simulink model "Control_model_10DOF_fin"  (R2016b)
settings: Solver=FixedStepAuto  StartTime=0.0  StopTime=10  FixedStep=0.0001  RelTol=1e-3
InitFcn:
  | Initialisation_ctr_10DOF_fin
values from neighbouring files (symbols this model uses):
  COM_Parameters = [-lpelvis/2;r2;0]    [Initialisation_ctr_10DOF_fin.m]
  DH_Parameters = [hfoot 0 ... (first row only)    [Initialisation_ctr_10DOF_fin.m]
  dTrunk = trunklbd(3)    [Initialisation_ctr_10DOF_fin.m]
  dxFootSM = dxFoot    [Initialisation_ctr_10DOF_fin.m]
  dxTrunk = 0.1    [Initialisation_ctr_10DOF_fin.m]
  Foot_Parameters = [0;-(lFoot/2-lHeel);0]    [Initialisation_ctr_10DOF_fin.m]
  HAA2HEE = [0; 0; 0.001]    [Initialisation_ctr_10DOF_fin.m]
  HEE2HFE = 0.5*[0.2; 0; 0]    [Initialisation_ctr_10DOF_fin.m]
  height_vrp = CoM_position(1)    [Initialisation_ctr_10DOF_fin.m]
  hTrunk = trunklbd(1)    [Initialisation_ctr_10DOF_fin.m]
  initial_CoM_position = R*CoM_position    [Initialisation_ctr_10DOF_fin.m]
  initial_CoM_velocity = [0;0;0]    [Initialisation_ctr_10DOF_fin.m]
  initial_left_foot = [0;0;-stance_width/2]    [Initialisation_ctr_10DOF_fin.m]
  initial_right_foot = [0;0;stance_width/2]    [Initialisation_ctr_10DOF_fin.m]
  initial_RorL = 0    [Initialisation_ctr_10DOF_fin.m]
  jointsinitial = [9;-15;6;0;0;6;-15;9]/180*pi    [Initialisation_ctr_10DOF_fin.m]
  K_DCM = 4.3*[1 0 0 ... (first row only)    [Initialisation_ctr_10DOF_fin.m]
  kD_left = mbody*[0.95 0 0 0 ... (first row only)    [Initialisation_ctr_10DOF_fin.m]
  kD_right = mbody*[0.12 0 0 0 ... (first row only)    [Initialisation_ctr_10DOF_fin.m]
  kI_left = mbody*[35 0 0 0 ... (first row only)    [Initialisation_ctr_10DOF_fin.m]
  kI_right = mbody*[38.2 0 0 0 ... (first row only)    [Initialisation_ctr_10DOF_fin.m]
  kP_left = mbody*[75 0 0 0 ... (first row only)    [Initialisation_ctr_10DOF_fin.m]
  kP_right = mbody*[5.6 0 0 0 ... (first row only)    [Initialisation_ctr_10DOF_fin.m]
  Lenght = [lShank;lThigh]    [Initialisation_ctr_10DOF_fin.m]
  lFootSM = lFoot    [Initialisation_ctr_10DOF_fin.m]
  lpelvis = wPelvis    [Initialisation_ctr_10DOF_fin.m]
  mass = mbody    (= 60)    [Initialisation_ctr_10DOF_fin.m]
  Masses = [mThigh; mShank; mTrunk]    [Initialisation_ctr_10DOF_fin.m]
  nb_step = 4    [Initialisation_ctr_10DOF_fin.m]
  nb_step_pattern = 20    [Initialisation_ctr_10DOF_fin.m]
  Pelvis_Parameters = [-lpelvis/2;hTrunk/2;0]    [Initialisation_ctr_10DOF_fin.m]
  stance_width = lpelvis    [Initialisation_ctr_10DOF_fin.m]
  stride_lenght = 0.50    (= 0.5)    [Initialisation_ctr_10DOF_fin.m]
  T_DS = time_DS    (= 0.4)    [Initialisation_ctr_10DOF_fin.m]
  T_IT = time_DS    (= 0.4)    [Initialisation_ctr_10DOF_fin.m]
  T_SS = time_swing    (= 1.6)    [Initialisation_ctr_10DOF_fin.m]
  time_DS = (time_stance-time_swing)/2    (= 0.4)    [Initialisation_ctr_10DOF_fin.m]
  time_stance = 60/100*time_stride    (= 2.4)    [Initialisation_ctr_10DOF_fin.m]
  time_step = time_stride/2    (= 2)    [Initialisation_ctr_10DOF_fin.m]
  time_swing = 40/100*time_stride    (= 1.6)    [Initialisation_ctr_10DOF_fin.m]
  validity_angle = [-20*pi/180 20*pi/180 ... (first row only)    [Initialisation_ctr_10DOF_fin.m]
  wTrunk = trunklbd(2)    [Initialisation_ctr_10DOF_fin.m]
  x4CoM = CoM_position(1)-XR4(1)    [Initialisation_ctr_10DOF_fin.m]
undefined symbols (not defined in the file or in its folder): dsegment, hFoot, l, lFoot, omega0_x, omega0_z, rho, wPelvis, X, Xp_x, Xp_z, Y, Z
undefined symbols (not defined in the file): k_grf, lShankSM, lThighSM, mShank, mThigh
libraries: nesl_utility x247, sm_lib x215, dspindex x12, FootPlacementLibrary x8, dspsigops x4, dspswit3 x1
(part 18 of 18)

== stateflow chart Control_model_10DOF_fin/Time//State Machine/Chart ==
  state DS_Transfert_Left
    entry: State=4;
    RorL=true;
  state Initial_Transfert_Right
    entry: State=1;
    RorL=false;
  state SS_Left_Swing
    entry: State=2;
    RorL=false;
  state Finish_Left_swing
    entry: State=3;
    RorL=false;
  state Stance
    entry: State=0;
  state Initial_Transfert_Left
    entry: State=1;
    RorL=true;
  state SS_Right_Swing
    entry: State=2;
    RorL=true;
  state DS_Transfert_Right
    entry: State=4;
    RorL=false;
  state Finish_Right_swing
    entry: State=3;
    RorL=true;
  DS_Transfert_Right -> SS_Left_Swing : [t>=T_DS]
  SS_Left_Swing -> DS_Transfert_Left [order 1] : [t>=T_SS && L_contact==1]
  Stance -> Initial_Transfert_Right [order 1] : [initial_RorL==0]
  DS_Transfert_Left -> SS_Right_Swing : [t>=T_DS]
  Finish_Left_swing -> DS_Transfert_Left : [L_contact==1]
  Initial_Transfert_Right -> SS_Left_Swing : [t>=T_IT]
  SS_Left_Swing -> Finish_Left_swing [order 2] : [t>=T_SS && L_contact==0]
  (default) -> Stance
  Stance -> Initial_Transfert_Left [order 2] : [initial_RorL==1]
  SS_Right_Swing -> DS_Transfert_Right [order 1] : [t>=T_SS && R_contact==1]
  Initial_Transfert_Left -> SS_Right_Swing : [t>=T_IT]
  SS_Right_Swing -> Finish_Right_swing [order 2] : [t>=T_SS && R_contact==0]
  Finish_Right_swing -> DS_Transfert_Right : [R_contact==1]
  data: t input; R_contact input; initial_RorL parameter; L_contact input; State output; RorL output boolean size=1; T_DS parameter; T_SS parameter; T_IT parameter

== matlab function Control_model_10DOF_fin/Trajectory generator/DCM trajectory/DS/DCM estimate fin ==
  data: r_vrp input double size=3; DCM_position output double size=3; DCM_velocity output double size=3; r_DCM input double size=3; time_stance parameter double size=1; height_vrp parameter double size=1; time input double size=1
 function [DCM_position,DCM_velocity] = DCM_trajectory_generator_DS(r_vrp,r_DCM,time_stance, height_vrp,time)

%gravity
g=9.81;

% r_vrp(2)=r_vrp(2)/2;
% r_DCM(2)=r_DCM(2)/2;

%% DCM Trajectory

DCM_position=r_vrp+exp(sqrt(g/height_vrp)*(time-time_stance))*(r_DCM-r_vrp);
DCM_velocity=sqrt(g/height_vrp)*exp(sqrt(g/height_vrp)*(time-time_stance))*(r_DCM-r_vrp);

== matlab function Control_model_10DOF_fin/Trajectory generator/DCM trajectory/DS/DCM_points_position ==
  data: feet_positions input double; r_vrp output double size=3*(nb_step-1); r_DCM output double size=3*(nb_step-2); height_vrp parameter size=1; time_step parameter size=1; nb_step parameter size=1; Foot_Parameters parameter
function [r_vrp,r_DCM] =  Point_positions(feet_positions,height_vrp, time_step,nb_step,Foot_Parameters )

for i=1:3:length(feet_positions)
    feet_positions(i:(i+2))=feet_positions(i:(i+2));%+Foot_Parameters;
end

%gravity
g=9.81;

r_vrp=zeros(3*(nb_step-1),1);
r_DCM=zeros(3*(nb_step-2),1);

%Virtual Repellent Point position
for i=1:(nb_step-1)
    r_vrp((3*(i-1)+1):(3*i),1)=feet_positions((3*(i)+1):(3*(i+1)),1)+[0;height_vrp;0];
end

%final DCM position
r_DCM((3*((nb_step-2)-1)+1):(3*(nb_step-2)),1)=r_vrp((3*(nb_step-2)+1):(3*(nb_step-1)),1);

%%DCM point creation
for i=nb_step-3:-1:1
    r_DCM(3*(i-1)+1:(3*i),1)=r_vrp(3*(i)+1:(3*(i+1)),1)+exp(-sqrt(g/height_vrp)*time_step)*(r_DCM(3*(i)+1:(3*(i+1)),1)-r_vrp((3*(i)+1):(3*(i+1))));
end

== matlab function Control_model_10DOF_fin/Trajectory generator/DCM trajectory/DS/MATLAB Function ==
  data: DCM_position_ini input; DCM_position output; DCM_velocity_ini input; DCM_position_fin input; DCM_velocity_fin input; DCM_velocity output; time input; time_DS parameter size=1
function [DCM_position,DCM_velocity] = Polynomial_interpolation(DCM_position_ini,DCM_velocity_ini,DCM_position_fin,DCM_velocity_fin,time, time_DS)

P=[2/time_DS^3 1/time_DS^2 -2/time_DS^3 1/time_DS^2;
    -3/time_DS^2 -2/time_DS 3/time_DS^2 -1/time_DS;
    0 1 0 0;
    1 0 0 0];
P=P*[DCM_position_ini';
    DCM_velocity_ini';
    DCM_position_fin';
    DCM_velocity_fin'];

 T=[time^3 time^2 time 1;
     3*time^2 2*time 1 0];
 
 Res=T*P;
 
 DCM_position=[Res(1,1);Res(1,2);Res(1,3)];
 DCM_velocity=[Res(2,1);Res(2,2);Res(2,3)];

end

== matlab function Control_model_10DOF_fin/Trajectory generator/DCM trajectory/Finish_swing_phase//SS/DCM trajectory generator ==
  data: r_vrp input double size=3; DCM_position output double size=3; DCM_velocity output double size=3; r_DCM input double size=3; time_stance parameter double size=1; height_vrp parameter double size=1; time input double size=1
function [DCM_position,DCM_velocity] = DCM_trajectory_generator(r_vrp,r_DCM,time_stance, height_vrp,time)

%gravity
g=9.81;

% r_vrp(2)=r_vrp(2)/2;
% r_DCM(2)=r_DCM(2)/2;

%% DCM Trajectory

DCM_position=r_vrp+exp(sqrt(g/height_vrp)*(time-time_stance))*(r_DCM-r_vrp);
DCM_velocity=sqrt(g/height_vrp)*exp(sqrt(g/height_vrp)*(time-time_stance))*(r_DCM-r_vrp);

== matlab function Control_model_10DOF_fin/Trajectory generator/DCM trajectory/Finish_swing_phase//SS/DCM_points_position ==
  data: feet_positions input double; r_vrp output double size=3*(nb_step-1); r_DCM output double size=3*(nb_step-2); height_vrp parameter size=1; time_step parameter size=1; nb_step parameter size=1; Foot_Parameters parameter
function [r_vrp,r_DCM] =  Point_positions(feet_positions,height_vrp, time_step,nb_step,Foot_Parameters )

for i=1:3:length(feet_positions)
    feet_positions(i:(i+2))=feet_positions(i:(i+2));%+Foot_Parameters;
end

%gravity
g=9.81;

r_vrp=zeros(3*(nb_step-1),1);
r_DCM=zeros(3*(nb_step-2),1);

%Virtual Repellent Point position
for i=1:(nb_step-1)
    r_vrp((3*(i-1)+1):(3*i),1)=feet_positions((3*(i)+1):(3*(i+1)),1)+[0;height_vrp;0];
end

%final DCM position
r_DCM((3*((nb_step-2)-1)+1):(3*(nb_step-2)),1)=r_vrp((3*(nb_step-2)+1):(3*(nb_step-1)),1);

%%DCM point creation
for i=nb_step-3:-1:1
    r_DCM(3*(i-1)+1:(3*i),1)=r_vrp(3*(i)+1:(3*(i+1)),1)+exp(-sqrt(g/height_vrp)*time_step)*(r_DCM(3*(i)+1:(3*(i+1)),1)-r_vrp((3*(i)+1):(3*(i+1))));
end

== matlab function Control_model_10DOF_fin/Trajectory generator/DCM trajectory/Initial_Transfert/DCM_estimate_fin/DCM trajectory generator ==
  data: r_vrp input double size=3; DCM_position output double size=3; DCM_velocity output double size=3; r_DCM input double size=3; time_stance parameter double size=1; height_vrp parameter double size=1; time input double size=1
 function [DCM_position,DCM_velocity] = DCM_trajectory_generator_DS(r_vrp,r_DCM,time_stance, height_vrp,time)

%gravity
g=9.81;

% r_vrp(2)=r_vrp(2)/2;
% r_DCM(2)=r_DCM(2)/2;

%% DCM Trajectory

DCM_position=r_vrp+exp(sqrt(g/height_vrp)*(time-time_stance))*(r_DCM-r_vrp);
DCM_velocity=sqrt(g/height_vrp)*exp(sqrt(g/height_vrp)*(time-time_stance))*(r_DCM-r_vrp);

== matlab function Control_model_10DOF_fin/Trajectory generator/DCM trajectory/Initial_Transfert/DCM_points_position ==
  data: feet_positions input double; r_vrp output double size=3*(nb_step-1); r_DCM output double size=3*(nb_step-2); height_vrp parameter size=1; time_step parameter size=1; nb_step parameter size=1; Foot_Parameters parameter
function [r_vrp,r_DCM] =  Point_positions(feet_positions,height_vrp, time_step,nb_step,Foot_Parameters )

for i=1:3:length(feet_positions)
    feet_positions(i:(i+2))=feet_positions(i:(i+2));%+Foot_Parameters;
end

%gravity
g=9.81;

r_vrp=zeros(3*(nb_step-1),1);
r_DCM=zeros(3*(nb_step-2),1);

%Virtual Repellent Point position
for i=1:(nb_step-1)
    r_vrp((3*(i-1)+1):(3*i),1)=feet_positions((3*(i)+1):(3*(i+1)),1)+[0;height_vrp;0];
end

%final DCM position
r_DCM((3*((nb_step-2)-1)+1):(3*(nb_step-2)),1)=r_vrp((3*(nb_step-2)+1):(3*(nb_step-1)),1);

%%DCM point creation
for i=nb_step-3:-1:1
    r_DCM(3*(i-1)+1:(3*i),1)=r_vrp(3*(i)+1:(3*(i+1)),1)+exp(-sqrt(g/height_vrp)*time_step)*(r_DCM(3*(i)+1:(3*(i+1)),1)-r_vrp((3*(i)+1):(3*(i+1))));
end

== matlab function Control_model_10DOF_fin/Trajectory generator/DCM trajectory/Initial_Transfert/MATLAB Function ==
  data: DCM_position_ini input; DCM_position output; DCM_velocity_ini input; DCM_position_fin input; DCM_velocity_fin input; DCM_velocity output; time input; T_IT parameter size=1
function [DCM_position,DCM_velocity] = Polynomial_interpolation(DCM_position_ini,DCM_velocity_ini,DCM_position_fin,DCM_velocity_fin,time, T_IT)

P=[2/T_IT^3 1/T_IT^2 -2/T_IT^3 1/T_IT^2;
    -3/T_IT^2 -2/T_IT 3/T_IT^2 -1/T_IT;
    0 1 0 0;
    1 0 0 0];
P=P*[DCM_position_ini';
    DCM_velocity_ini';
    DCM_position_fin';
    DCM_velocity_fin'];

 T=[time^3 time^2 time 1;
     3*time^2 2*time 1 0];
 
 Res=T*P;
 
 DCM_position=[Res(1,1);Res(1,2);Res(1,3)];
 DCM_velocity=[Res(2,1);Res(2,2);Res(2,3)];

end

== matlab function Control_model_10DOF_fin/Trajectory generator/Enabled and Triggered Subsystem 1/Feet Pattern generator/Pattern creator ==
  data: swing_foot_position input size=[3 1]; stance_foot_position input double size=3; feet_positions output double size=3*(nb_step_pattern); RorL input size=1; nb_step_pattern parameter single size=1; stride_lenght parameter double size=1; stance_width parameter single size=1
  function feet_positions  = pattern_creator(swing_foot_position,stance_foot_position,RorL,nb_step_pattern,stride_lenght,stance_width)

feet_positions=zeros(3*(nb_step_pattern),1);


feet_positions(1:3,1)=swing_foot_position(:);
feet_positions(4:6,1)=stance_foot_position(:);
if RorL==true
    feet_positions(7:9,1)=stance_foot_position(:)+[stride_lenght/2;0;stance_width];
    if nb_step_pattern==4
        feet_positions(10:12,1)=feet_positions(7:9,1)+[0;0;-stance_width];
    end
else
    feet_positions(7:9,1)=stance_foot_position(:)+[stride_lenght/2;0;-stance_width];
    if nb_step_pattern==4
        feet_positions(10:12,1)=feet_positions(7:9,1)+[0;0;stance_width];
    end
end

if nb_step_pattern>4
    for i=4:nb_step_pattern-1
        if i==nb_step_pattern
            feet_positions((3*(i-1)+1):(3*i),1)=feet_positions((3*(i-3)+1):(3*(i-2)),1)+[stride_lenght/2;0;0];
        else
            feet_positions((3*(i-1)+1):(3*i),1)=feet_positions((3*(i-3)+1):(3*(i-2)),1)+[stride_lenght;0;0];
        end
        if i~=nb_step_pattern
            if i+1==nb_step_pattern
                feet_positions((3*i+1):(3*(i+1)),1)=feet_positions((3*(i-2)+1):(3*(i-1)),1)+[stride_lenght/2;0;0];
            else
                feet_positions((3*i+1):(3*(i+1)),1)=feet_positions((3*(i-2)+1):(3*(i-1)),1)+[stride_lenght;0;0];
            end
        end
    end
end

== matlab function Control_model_10DOF_fin/Trajectory generator/Enabled and Triggered Subsystem 1/initial position1/Left/MATLAB Function ==
  data: T input; X output
function X = fcn(T)

X=T(1:3,4);
X(2)=0;

== matlab function Control_model_10DOF_fin/Trajectory generator/Enabled and Triggered Subsystem 1/initial position1/Left/MATLAB Function1 ==
  data: T input; X output
function X = fcn(T)

X=T(1:3,4);
X(2)=0;

== matlab function Control_model_10DOF_fin/Trajectory generator/Enabled and Triggered Subsystem 1/initial position1/Right/MATLAB Function ==
  data: T input; X output
function X = fcn(T)

X=T(1:3,4);
X(2)=0;

== matlab function Control_model_10DOF_fin/Trajectory generator/Enabled and Triggered Subsystem 1/initial position1/Right/MATLAB Function1 ==
  data: T input; X output
function X = fcn(T)

X=T(1:3,4);
X(2)=0;

== matlab function Control_model_10DOF_fin/Trajectory generator/Enabled and Triggered Subsystem 1/initial position2/Left/MATLAB Function ==
  data: T input; X output
function X = fcn(T)

X=T(1:3,4);
X(2)=0;

== matlab function Control_model_10DOF_fin/Trajectory generator/Enabled and Triggered Subsystem 1/initial position2/Left/MATLAB Function1 ==
  data: T input; X output
function X = fcn(T)

X=T(1:3,4);
X(2)=0;

== matlab function Control_model_10DOF_fin/Trajectory generator/Enabled and Triggered Subsystem 1/initial position2/Right/MATLAB Function ==
  data: T input; X output
function X = fcn(T)

X=T(1:3,4);
X(2)=0;

== matlab function Control_model_10DOF_fin/Trajectory generator/Enabled and Triggered Subsystem 1/initial position2/Right/MATLAB Function1 ==
  data: T input; X output
function X = fcn(T)

X=T(1:3,4);
X(2)=0;

== matlab function Control_model_10DOF_fin/Trajectory generator/Hip trajectory2/DS/Hip trajectory ==
  data: current_time input; hip_angle_des output double size=1; time_DS parameter double size=1
function hip_angle_des= hip_trajectory(current_time, time_DS)


%% knee trajectory

knee_angle_ini=0;
knee_angle_fin=-3.3*pi/180;

slope_ini=0; 
slope_fin=0;

% current_time=current_time;
% 
% knee_angle_des=knee_angle_ini+slope_ini*current_time+(3*(knee_angle_fin-knee_angle_ini)-2*slope_ini-slope_fin)*(current_time)^2+(2*(knee_angle_ini-knee_angle_fin)+slope_ini+slope_fin)*(current_time)^3;

P=[2/(time_DS)^3 1/(time_DS)^2 -2/(time_DS)^3 1/(time_DS)^2;
    -3/(time_DS)^2 -2/(time_DS) 3/(time_DS)^2 -1/(time_DS);
    0 1 0 0;
    1 0 0 0];
P=P*[knee_angle_ini;
    slope_ini;
    knee_angle_fin;
    slope_fin];

 time_DS=[current_time^3 current_time^2 current_time 1;
     3*current_time^2 2*current_time 1 0];
 
 Res=time_DS*P;
 
 hip_angle_des=Res(1,1);

== matlab function Control_model_10DOF_fin/Trajectory generator/Hip trajectory2/Initial_Transfert/Hip trajectory ==
  data: current_time input; time_DS parameter double size=1; hip_angle_des output double size=1
function hip_angle_des= hip_trajectory(current_time, time_DS)


%% knee trajectory

knee_angle_ini=0;
knee_angle_fin=-3.3*pi/180;

slope_ini=0; 
slope_fin=0;

% current_time=current_time;
% 
% knee_angle_des=knee_angle_ini+slope_ini*current_time+(3*(knee_angle_fin-knee_angle_ini)-2*slope_ini-slope_fin)*(current_time)^2+(2*(knee_angle_ini-knee_angle_fin)+slope_ini+slope_fin)*(current_time)^3;

P=[2/(time_DS)^3 1/(time_DS)^2 -2/(time_DS)^3 1/(time_DS)^2;
    -3/(time_DS)^2 -2/(time_DS) 3/(time_DS)^2 -1/(time_DS);
    0 1 0 0;
    1 0 0 0];
P=P*[knee_angle_ini;
    slope_ini;
    knee_angle_fin;
    slope_fin];

 T=[current_time^3 current_time^2 current_time 1;
     3*current_time^2 2*current_time 1 0];
 
 Res=T*P;
 
 hip_angle_des=Res(1,1);

== matlab function Control_model_10DOF_fin/Trajectory generator/Hip trajectory2/SS/Subsystem2/Subsystem/Hip trajectory ==
  data: current_time input; time_swing parameter double size=1; hip_angle_des output double size=1
function hip_angle_des= hip_trajectory(current_time, time_swing)


%% knee trajectory

knee_angle_ini=-3.3*pi/180;
knee_angle_fin=0;

slope_ini=0; 
slope_fin=0;

% current_time=current_time;
% 
% knee_angle_des=knee_angle_ini+slope_ini*current_time+(3*(knee_angle_fin-knee_angle_ini)-2*slope_ini-slope_fin)*(current_time)^2+(2*(knee_angle_ini-knee_angle_fin)+slope_ini+slope_fin)*(current_time)^3;

P=[2/(time_swing/2)^3 1/(time_swing/2)^2 -2/(time_swing/2)^3 1/(time_swing/2)^2;
    -3/(time_swing/2)^2 -2/(time_swing/2) 3/(time_swing/2)^2 -1/(time_swing/2);
    0 1 0 0;
    1 0 0 0];
P=P*[knee_angle_ini;
    slope_ini;
    knee_angle_fin;
    slope_fin];

 T=[current_time^3 current_time^2 current_time 1;
     3*current_time^2 2*current_time 1 0];
 
 Res=T*P;
 
 hip_angle_des=Res(1,1);

== matlab function Control_model_10DOF_fin/Trajectory generator/Subsystem1/SS/Swing foot trajectory ==
  data: Swing_foot_position_des output; foot_position_ini input; foot_position_fin input; time input double size=1; time_swing parameter double size=1
function Swing_foot_position_des  = Polynomial_interpolation(foot_position_ini,foot_position_fin,time, time_swing)

P=[2/(time_swing)^3 1/(time_swing)^2 -2/(time_swing)^3 1/(time_swing)^2;
    -3/(time_swing)^2 -2/(time_swing) 3/(time_swing)^2 -1/(time_swing);
    0 1 0 0;
    1 0 0 0];
P=P*[foot_position_ini';
    0 0 0;
    foot_position_fin';
    0 0 0];

 T=[time^3 time^2 time 1;
     3*time^2 2*time 1 0];
 
Res=T*P;
Swing_foot_position_des=Res(1,1:3).';
 

end

== matlab function Control_model_10DOF_fin/Trajectory generator/knee trajectory/DS/Left transfer/Swing leg trajectory1 ==
  data: current_time input; knee_angle_ini input; knee_angle_des output double size=1; time_DS parameter
function knee_angle_des    = knee_trajectory(current_time,knee_angle_ini,time_DS)


%% knee trajectory

knee_angle_fin=-30*pi/180;

slope_ini=0; 
slope_fin=0;

% current_time=current_time;
% 
% knee_angle_des=knee_angle_ini+slope_ini*current_time+(3*(knee_angle_fin-knee_angle_ini)-2*slope_ini-slope_fin)*(current_time)^2+(2*(knee_angle_ini-knee_angle_fin)+slope_ini+slope_fin)*(current_time)^3;


P=[2/(time_DS)^3 1/(time_DS)^2 -2/(time_DS)^3 1/(time_DS)^2;
    -3/(time_DS)^2 -2/(time_DS) 3/(time_DS)^2 -1/(time_DS);
    0 1 0 0;
    1 0 0 0];
P=P*[knee_angle_ini;
    slope_ini;
    knee_angle_fin;
    slope_fin];

 T=[current_time^3 current_time^2 current_time 1;
     3*current_time^2 2*current_time 1 0];
 
 Res=T*P;
 
 knee_angle_des=Res(1,1);

== matlab function Control_model_10DOF_fin/Trajectory generator/knee trajectory/DS/Right transfer/Swing leg trajectory1 ==
  data: current_time input; knee_angle_ini input; knee_angle_des output double size=1; time_DS parameter
function knee_angle_des    = knee_trajectory(current_time,knee_angle_ini,time_DS)


%% knee trajectory

knee_angle_fin=-30*pi/180;

slope_ini=0; 
slope_fin=0;

% current_time=current_time;
% 
% knee_angle_des=knee_angle_ini+slope_ini*current_time+(3*(knee_angle_fin-knee_angle_ini)-2*slope_ini-slope_fin)*(current_time)^2+(2*(knee_angle_ini-knee_angle_fin)+slope_ini+slope_fin)*(current_time)^3;


P=[2/(time_DS)^3 1/(time_DS)^2 -2/(time_DS)^3 1/(time_DS)^2;
    -3/(time_DS)^2 -2/(time_DS) 3/(time_DS)^2 -1/(time_DS);
    0 1 0 0;
    1 0 0 0];
P=P*[knee_angle_ini;
    slope_ini;
    knee_angle_fin;
    slope_fin];

 T=[current_time^3 current_time^2 current_time 1;
     3*current_time^2 2*current_time 1 0];
 
 Res=T*P;
 
 knee_angle_des=Res(1,1);

== matlab function Control_model_10DOF_fin/Trajectory generator/knee trajectory/SS/Left swing /Swing leg trajectory1 ==
  data: current_time input; knee_angle_ini input; knee_angle_des output double size=1; time_swing parameter
function knee_angle_des    = knee_trajectory(current_time,knee_angle_ini,time_swing)


%% knee trajectory

knee_angle_fin=-15*pi/180;

slope_ini=0; 
slope_fin=0;

% current_time=current_time;
% 
% knee_angle_des=knee_angle_ini+slope_ini*current_time+(3*(knee_angle_fin-knee_angle_ini)-2*slope_ini-slope_fin)*(current_time)^2+(2*(knee_angle_ini-knee_angle_fin)+slope_ini+slope_fin)*(current_time)^3;


P=[2/(time_swing)^3 1/(time_swing)^2 -2/(time_swing)^3 1/(time_swing)^2;
    -3/(time_swing)^2 -2/(time_swing) 3/(time_swing)^2 -1/(time_swing);
    0 1 0 0;
    1 0 0 0];
P=P*[knee_angle_ini;
    slope_ini;
    knee_angle_fin;
    slope_fin];

 T=[current_time^3 current_time^2 current_time 1;
     3*current_time^2 2*current_time 1 0];
 
 Res=T*P;
 
 knee_angle_des=Res(1,1);

== matlab function Control_model_10DOF_fin/Trajectory generator/knee trajectory/SS/Left swing /knee trajectory/Swing leg trajectory1 ==
  data: current_time input; knee_angle_ini input; knee_angle_des output double size=1; time_swing parameter
function knee_angle_des    = knee_trajectory(current_time,knee_angle_ini,time_swing)


%% knee trajectory

knee_angle_fin=-75*pi/180;

slope_ini=0; 
slope_fin=0;

% current_time=current_time;
% 
% knee_angle_des=knee_angle_ini+slope_ini*current_time+(3*(knee_angle_fin-knee_angle_ini)-2*slope_ini-slope_fin)*(current_time)^2+(2*(knee_angle_ini-knee_angle_fin)+slope_ini+slope_fin)*(current_time)^3;


P=[2/(time_swing/2)^3 1/(time_swing/2)^2 -2/(time_swing/2)^3 1/(time_swing/2)^2;
    -3/(time_swing/2)^2 -2/(time_swing/2) 3/(time_swing/2)^2 -1/(time_swing/2);
    0 1 0 0;
    1 0 0 0];
P=P*[knee_angle_ini;
    slope_ini;
    knee_angle_fin;
    slope_fin];

 T=[current_time^3 current_time^2 current_time 1;
     3*current_time^2 2*current_time 1 0];
 
 Res=T*P;
 
 knee_angle_des=Res(1,1);

== matlab function Control_model_10DOF_fin/Trajectory generator/knee trajectory/SS/Left swing /knee trajectory1/Swing leg trajectory1 ==
  data: current_time input; time_swing parameter double size=1; knee_angle_des output double size=1; knee_angle_ini input
function knee_angle_des    = knee_trajectory(current_time, time_swing, knee_angle_ini)


%% knee trajectory


knee_angle_fin=-15*pi/180;

slope_ini=0; 
slope_fin=0;

% current_time=current_time;
% 
% knee_angle_des=knee_angle_ini+slope_ini*current_time+(3*(knee_angle_fin-knee_angle_ini)-2*slope_ini-slope_fin)*(current_time)^2+(2*(knee_angle_ini-knee_angle_fin)+slope_ini+slope_fin)*(current_time)^3;


P=[2/(time_swing/2)^3 1/(time_swing/2)^2 -2/(time_swing/2)^3 1/(time_swing/2)^2;
    -3/(time_swing/2)^2 -2/(time_swing/2) 3/(time_swing/2)^2 -1/(time_swing/2);
    0 1 0 0;
    1 0 0 0];
P=P*[knee_angle_ini;
    slope_ini;
    knee_angle_fin;
    slope_fin];

 T=[current_time^3 current_time^2 current_time 1;
     3*current_time^2 2*current_time 1 0];
 
 Res=T*P;
 
 knee_angle_des=Res(1,1);

== matlab function Control_model_10DOF_fin/Trajectory generator/knee trajectory/SS/Right swing/Swing leg trajectory1 ==
  data: current_time input; knee_angle_ini input; knee_angle_des output double size=1; time_swing parameter
function knee_angle_des    = knee_trajectory(current_time,knee_angle_ini,time_swing)


%% knee trajectory

knee_angle_fin=-15*pi/180;

slope_ini=0; 
slope_fin=0;

% current_time=current_time;
% 
% knee_angle_des=knee_angle_ini+slope_ini*current_time+(3*(knee_angle_fin-knee_angle_ini)-2*slope_ini-slope_fin)*(current_time)^2+(2*(knee_angle_ini-knee_angle_fin)+slope_ini+slope_fin)*(current_time)^3;


P=[2/(time_swing)^3 1/(time_swing)^2 -2/(time_swing)^3 1/(time_swing)^2;
    -3/(time_swing)^2 -2/(time_swing) 3/(time_swing)^2 -1/(time_swing);
    0 1 0 0;
    1 0 0 0];
P=P*[knee_angle_ini;
    slope_ini;
    knee_angle_fin;
    slope_fin];

 T=[current_time^3 current_time^2 current_time 1;
     3*current_time^2 2*current_time 1 0];
 
 Res=T*P;
 
 knee_angle_des=Res(1,1);

== matlab function Control_model_10DOF_fin/Trajectory generator/knee trajectory/SS/Right swing/knee trajectory/Swing leg trajectory1 ==
  data: current_time input; knee_angle_ini input; knee_angle_des output double size=1; time_swing parameter
function knee_angle_des    = knee_trajectory(current_time,knee_angle_ini,time_swing)


%% knee trajectory

knee_angle_fin=-75*pi/180;

slope_ini=0; 
slope_fin=0;

% current_time=current_time;
% 
% knee_angle_des=knee_angle_ini+slope_ini*current_time+(3*(knee_angle_fin-knee_angle_ini)-2*slope_ini-slope_fin)*(current_time)^2+(2*(knee_angle_ini-knee_angle_fin)+slope_ini+slope_fin)*(current_time)^3;


P=[2/(time_swing/2)^3 1/(time_swing/2)^2 -2/(time_swing/2)^3 1/(time_swing/2)^2;
    -3/(time_swing/2)^2 -2/(time_swing/2) 3/(time_swing/2)^2 -1/(time_swing/2);
    0 1 0 0;
    1 0 0 0];
P=P*[knee_angle_ini;
    slope_ini;
    knee_angle_fin;
    slope_fin];

 T=[current_time^3 current_time^2 current_time 1;
     3*current_time^2 2*current_time 1 0];
 
 Res=T*P;
 
 knee_angle_des=Res(1,1);

== matlab function Control_model_10DOF_fin/Trajectory generator/knee trajectory/SS/Right swing/knee trajectory1/Swing leg trajectory1 ==
  data: current_time input; time_swing parameter double size=1; knee_angle_des output double size=1; knee_angle_ini input
function knee_angle_des    = knee_trajectory(current_time, time_swing, knee_angle_ini)


%% knee trajectory


knee_angle_fin=-15*pi/180;

slope_ini=0; 
slope_fin=0;

% current_time=current_time;
% 
% knee_angle_des=knee_angle_ini+slope_ini*current_time+(3*(knee_angle_fin-knee_angle_ini)-2*slope_ini-slope_fin)*(current_time)^2+(2*(knee_angle_ini-knee_angle_fin)+slope_ini+slope_fin)*(current_time)^3;


P=[2/(time_swing/2)^3 1/(time_swing/2)^2 -2/(time_swing/2)^3 1/(time_swing/2)^2;
    -3/(time_swing/2)^2 -2/(time_swing/2) 3/(time_swing/2)^2 -1/(time_swing/2);
    0 1 0 0;
    1 0 0 0];
P=P*[knee_angle_ini;
    slope_ini;
    knee_angle_fin;
    slope_fin];

 T=[current_time^3 current_time^2 current_time 1;
     3*current_time^2 2*current_time 1 0];
 
 Res=T*P;
 
 knee_angle_des=Res(1,1);
